simulink model "BiT_Template"  (R2025a)
settings: Solver=FixedStepDiscrete  StartTime=0.0  StopTime=Inf  FixedStep=0.005  RelTol=1e-3
StopFcn:
  | user_confirmed = true;
  | disp('Gestoppt?!')
  | 
  | % stop(t);
  | % delete(t);
  | 
  | %% Switch to Config Mode
  | %Tc3_AI.sysManager.ActivateConfiguration();
  | %
  | % Tc3_AI.SwitchToConfig('local')
  | %
  | % %save Solution
  | % Tc3_AI.SaveSolution();
  | %
  | % %% Close Aktive VS Instance
  | % Tc3_AI.closeVsInstance();
libraries: slpidlib x1
settings Model: SimulationMode=external  Creator=clemensm  LastModifiedBy=Lenard
settings OptimizationCC: LocalBlockOutputs=off
settings RTWCC: SystemTargetFile=TwinCatGrt.tlc  GenCodeOnly=on  GenerateMakefile=off  TemplateMakefile=tcgrt_msbuild.tmf  TargetLang=C++  Description=TwinCAT GRT Target
settings STFCustomTargetCC: SystemTargetFile=TwinCatGrt.tlc  TargetLangStandard=C++11 (ISO)  MultiwordLength=2048.0  DynamicStringBufferSize=256.0  ConcurrentExecutionCompliant=on  CombineOutputUpdateFcns=on  CodeInterfacePackaging=Reusable function  CPPClassGenCompliant=on  GRTInterface=off  GenerateAllocFcn=on  TcCom_DWorkReadOnly=on  TcProject_InstallPlcLibrary=off  TcProject_CLanguageStandard=Default  TcProject_PlcVarPrefixes=PVOID=p | BOOL=b | BOOL32=b | DATE=d | TIME_OF_DATE=td | TIME=t | LTIME=t | GUID=n  TcProject_PreferIntOverLong=off  TcPlcFb_OemLicenses=$<Project:OemLicenses>  TcCom_OutputCreateSymbols=on  TcCom_AccessLockState=Auto  TcProject_PublishTcUMx86=off  TcProject_PublishTcRTx64=on  TcPlcFb_ExtModeRtAllowExecutionCommands=off  TcCom_TcComWrapperFbProperties=off  TcProject_PublishTcOSARMv7M=off  TcCom_GroupIcon=$<TE140x:Icon>  TcCom_ModuleIcon=$<TE140x:Icon>  TcCom_ExecutionInfoParam=on  TcCom_CallerVerification=Default  TcProject_PublishTcRTx86=on  TcProject_CreateScopedEnums=Auto  TcCom_ExtModeRtWaitForStart=off  TcProject_TmxInstall=on  TcProject_Description=TwinCAT executable file, generated by TwinCAT $<ModuleGenerator:ProductId>  TcCom_ParametersReadOnly=off  TcCom_GroupDisplayName=$<GroupName>  TcProject_MaxVisibleArrayElements=200U  TcProject_ClassFactoryName=$<Project:Name>  TcCom_TcComWrapperFb=off  TcCom_UpdateExceptionHandling=CallerExceptions  TcProject_UseStaticStlString=off  TcCom_BlockIoReadOnly=on  TcCom_Legacy_ModuleBuildInfoParam=on  TcProject_UseCodeInfoExporter=on  TcProject_ProjectDir=C:\TwinCAT\3.1\CustomConfig\Modules\Ctrl_only  TcCom_ExtModeRtAllowForParameterChange=on  TcProject_GenerateStructDutsWithDefaultValues=Auto  TcProject_PublishTcOSx64=off  TcCom_OnlineChangeRestoreDataAreas=off  TcCom_BlockDiagramVariableAccess=AssignToParent  TcProject_LibraryCategories=$<VendorName>  TcProject_DeployRestart=off  TcProject_PublishTcOSARMv8A=off  TcProject_PublishPlatformtoolset=Auto  TcProject_UseIntrinsics=on  TcCom_ExecutionSequence=UpdateBeforeOutputMapping  TcCom_TcComWrapperFbPropertyMonitoring=NoMonitoring  TcProject_SignWithTwinCatCertificate=inherit default  TcProject_LowestCompatibleTcBuild=$<TwinCAT:Version:BUILD>  TcCom_StrictAccessLock=on  TcCom_ContStateDataAccess=Internal DataArea  TcCom_ExecutionInfoOutput=off  TcCom_OemLicenses=$<Project:OemLicenses>  TcCom_Generate=on  TcProject_ForceRebuildForPublish=off  TcProject_CppLanguageStandard=Default  TcProject_EnableNewPlatforms=off  TcCom_BlockDiagramDebugInfoExport=on  TcCom_StepSizeAdaptation=RequireMatchingTaskCycleTime  TcCom_InitExceptionHandling=CallerExceptions  TcProject_BuildWithWdk=inherit default  TcProject_VendorIcon=$<TE140x:Icon>  TcCom_InputReadOnly=off  TcCom_BlockIoDataAccess=Internal DataArea  TcProject_StaticStlStringCapacity=Auto  TcProject_ProductName=$<ModuleGenerator:ProductId> $<ModuleGenerator:Version:MAJOR.MINOR>  TcCom_DataStoreDataAccess=None  TcCom_InputInitValues=off  TcProject_IncrementVersion=Revision  TcProject_GenerateVsSolution=No  TcProject_Publish=on  TcProject_DataExchangeModulesVersion=$<ModuleGenerator:DataExchange:Version>  TcProject_BuildSystem=Auto  TcProject_Versioning=Versioned  TcCom_ExtendSignalResolution=on  TcCom_ResolveMaskedSubsystems=on  TcProject_SignTwinCatCertName=MCI_2024_OEM.tccert  TcProject_PublishParallel=on  TcPlcFb_Generate=off  TcCom_BlockIoCreateSymbols=on  TcCom_DWorkDataAccess=Internal DataArea  TcProject_VersionSrc=$<LatestTMFile>  TcProject_Verbosity=Normal  TcPlcFb_MonitorExecutionTime=off  TcPlcFb_UpdateExceptionHandling=CallerExceptions  TcProject_CoderCppNamespace=coder  TcCom_DWorkCreateSymbols=on  TcPlcFb_ExtModeRtWaitForStart=off  TcCom_AllowDataAreaForSharedData=off  TcCom_ParametersDataAccess=Internal DataArea  TcProject_UseTmxExtension=Auto  TcProject_DrvFileVersion=$<VersionFromFile>  TcCom_GlobalParamDefaultSharing=Define  TcCom_ParametersInitValues=on  TcCom_OutputReadOnly=on  TcProject_GeneratePlcLibrary=off  TcCom_ContStateCreateSymbols=on  TcCom_MonitorExecutionTime=off  TcProject_PublishTcUMx64=off  TcProject_PreferToolArchitectureX64=on  TcCom_GroupName=TE140x|Simulink Modules  TcCom_BlockDiagramExport=on  TcCom_ExecuteModelCode=on  TcProject_CreateUniqueEnumItemNames=off  TcProject_PublishConfiguration=Release  TcCom_ExtModeRtAllowExecutionCommands=on  TcProject_PublishTcOSARMv7A=off  TcProject_UseDescriptorCodeType=on  TcCom_ContStateReadOnly=on  TcCom_ParametersCreateSymbols=on  TcPlcFb_InitExceptionHandling=CallerExceptions  TcCom_ModuleCaller=CyclicTask  TcCom_OnlineChange=off  TcCom_InputDataAccess=Input Destination DataArea  TcCom_InputCreateSymbols=on  TcProject_DrvProductVersion=$<DrvFileVersion>  TcPlcFb_ExtModeRtAllowForParameterChange=off  TcCom_VariableSymbolMapping=Identical  TcCom_DataStoreReadOnly=off  TcCom_OriginalIoBlockNames=off  TcProject_UseCodeDescriptor=on  TcProject_VendorName=TE140x Module Vendor  TcProject_Copyright=Copyright $<VendorName> $<LocalDateTime:%Y>  TcProject_Generate=on  TcCom_DataStoreCreateSymbols=on  TcCom_OutputDataAccess=Output Source DataArea  TcProject_LibCatPath=$<Project:Dir>\$<Project:Name>.libcat.xml  TcProject_UseNativeBlockDiagramExport=off  TcProject_UseDataExchangeModules=off
settings GRTTargetCC: ExtMode=on  ExtModeMexFile=TcExtModeClient  MultiInstanceErrorCode=None  TargetLangStandard=C++11 (ISO)  ParMdlRefBuildCompliant=off  CompOptLevelCompliant=off  MatFileLogging=off  CodeInterfacePackaging=Reusable function  GenerateAllocFcn=on  UseToolchainInfoCompliant=off

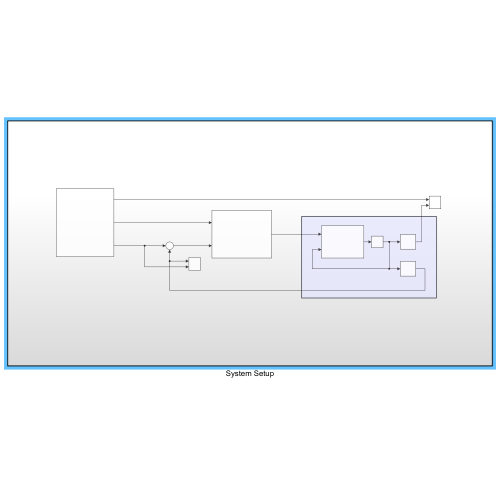
[thumbnail: Simulink's stored preview of the top-level diagram]
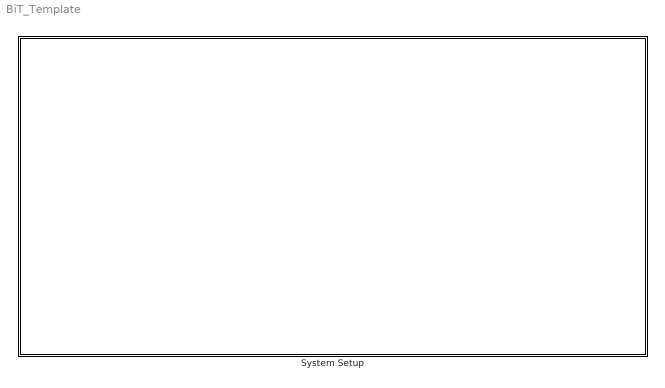
== system BiT_Template ==
  System Setup : Subsystem

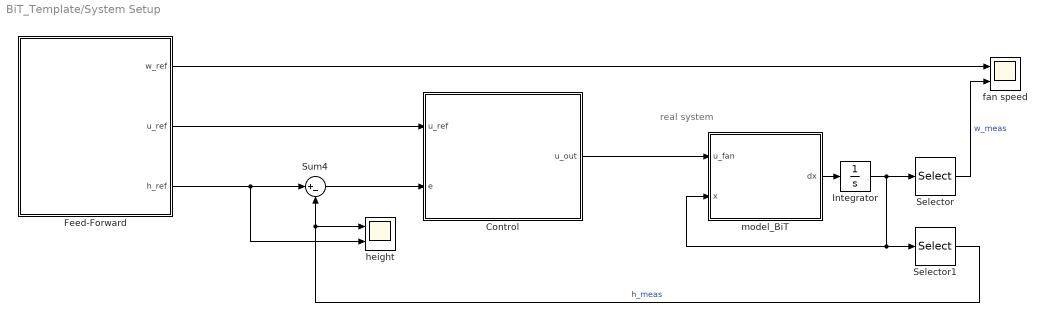
== system BiT_Template/System Setup ==
  note: real system
  Control : Subsystem
  Feed-Forward : Subsystem
  Integrator : Integrator
  Selector : Selector  InputPortWidth=3  IndexOptions=Index vector (dialog)  Indices=3  OutputSizes=1
  Selector1 : Selector  InputPortWidth=3  IndexOptions=Index vector (dialog)  Indices=1  OutputSizes=1
  Sum4 : Sum  Inputs=|+-
  fan speed : Scope  NumInputPorts=2
      settings: TimeSpan=60  ActiveDisplayYMinimum=4277  ActiveDisplayYMaximum=4777
  height : Scope  NumInputPorts=2
      settings: TimeSpan=60  ActiveDisplayYMinimum=0.11937  ActiveDisplayYMaximum=0.40562  DataLoggingVariableName=ScopeData2
  model_BiT : MATLAB Function  TreatAsAtomicUnit=on
  wires:
  Selector1/1 -> height/1, Sum4/2  "h_meas"
  Selector/1 -> fan speed/2  "w_meas"
  model_BiT/1(dx) -> Integrator/1
  Integrator/1 -> Selector/1, Selector1/1, model_BiT/2(x)
  Feed-Forward/3(h_ref) -> height/2, Sum4/1
  Feed-Forward/1(w_ref) -> fan speed/1
  Feed-Forward/2(u_ref) -> Control/1(u_ref)
  Sum4/1 -> Control/2(e)
  Control/1(u_out) -> model_BiT/1(u_fan)

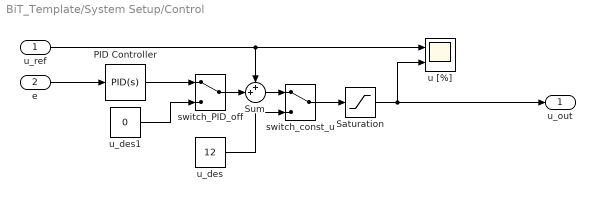
== system BiT_Template/System Setup/Control ==
  u_ref : Inport
  e : Inport  Port=2
  PID Controller : slpidlib/PID Controller  Controller=PID  Form=Parallel  TimeDomain=Continuous-time  UseExternalTs=off  SampleTime=-1  IntegratorMethod=Forward Euler  FilterMethod=Forward Euler  ControllerParametersSource=internal  P=1  I=1  UseKiTs=off  D=0  UseExternalDerivativeSource=off  N=100  UseFilter=on  TunerSelectOption=Transfer Function Based (PID Tuner App)  InitialConditionSource=internal  InitialConditionForIntegrator=0  InitialConditionForFilter=0  DifferentiatorICPrevScaledInput=0  ExternalReset=none  TrackingMode=off  Kt=1  LimitOutput=off  SatLimitsSource=internal  UpperSaturationLimit=inf  LowerSaturationLimit=-inf  LinearizeAsGain=on  AntiWindupMode=none  Kb=1  LimitIntegrator=off  UpperIntegratorSaturationLimit=inf  LowerIntegratorSaturationLimit=-inf  POutMin=[]  POutMax=[]  IOutMin=[]  IOutMax=[]  DOutMin=[]  DOutMax=[]  NOutMin=[]  NOutMax=[]  SumOutMin=[]  SumOutMax=[]  SaturationOutMin=[]  SaturationOutMax=[]  PParamMin=[]  PParamMax=[]  IParamMin=[]  IParamMax=[]  DParamMin=[]  DParamMax=[]  NParamMin=[]  NParamMax=[]  KbParamMin=[]  KbParamMax=[]  KtParamMin=[]  KtParamMax=[]  KbOutMin=[]  KbOutMax=[]  KtOutMin=[]  KtOutMax=[]  IntegratorOutMin=[]  IntegratorOutMax=[]  FilterOutMin=[]  FilterOutMax=[]  SumI1OutMin=[]  SumI1OutMax=[]  SumI2OutMin=[]  SumI2OutMax=[]  SumI3OutMin=[]  SumI3OutMax=[]  SumI4OutMin=[]  SumI4OutMax=[]  SumDOutMin=[]  SumDOutMax=[]  DifferentiatorOutMin=[]  DifferentiatorOutMax=[]  FilterDiffOutCoefMin=[]  FilterDiffOutCoefMax=[]  ReciprocalOutMin=[]  ReciprocalOutMax=[]  SumDenOutMin=[]  SumDenOutMax=[]  SumNumOutMin=[]  SumNumOutMax=[]  DivideOutMin=[]  DivideOutMax=[]  UdiffTsProdOutMin=[]  UdiffTsProdOutMax=[]  NTsProdOutMin=[]  NTsProdOutMax=[]  UintegralTsProdOutMin=[]  UintegralTsProdOutMax=[]  UngainTsProdOutMin=[]  UngainTsProdOutMax=[]  ClampingZeroOutDataTypeStr=Inherit: Inherit via back propagation  ClampingZeroOutMin=[]  ClampingZeroOutMax=[]  FilterDenConstantOutDataTypeStr=Inherit: Inherit via back propagation  FilterDenConstantOutMin=[]  FilterDenConstantOutMax=[]  PCopyOutDataTypeStr=Inherit: Inherit via back propagation  PCopyOutMin=[]  PCopyOutMax=[]  NCopyOutDataTypeStr=Inherit: Inherit via back propagation  NCopyOutMin=[]  NCopyOutMax=[]  IntegratorContinuousStateAttributes=''  IntegratorStateMustResolveToSignalObject=off  IntegratorRTWStateStorageClass=Auto  FilterContinuousStateAttributes=''  FilterStateMustResolveToSignalObject=off  FilterRTWStateStorageClass=Auto  ParallelPVariant=InternalParameters  IdealPVariant=Disabled  IVariant=InternalParameters  DVariant=InternalParameters  IntegratorVariant=Continuous  SatVariant=Disabled  AWVariant=Passthrough  PCopyVariant=Disabled  TRVariant=Disabled  FdbkBlocksVariant=Forward  IdealPFdbkVariant=Disabled  SatFdbkVariant=Disabled  DerivativeFilterVariant=ContFilter  NVariant=InternalParameters  NCopyVariant=Disabled  FilterICVariant=InternalICsFilter  IntegratorICVariant=InternalICs  ExternalResetVariant=Disabled  TRSumVariant=Passthrough  SumFdbkVariant=Disabled  SumVariant=Sum_PID  TsampFilterVariant=InternalTs  TsampNgainVariant=Passthrough  TsampIntegralVariant=Disabled_SignalSpec  ExternalSaturationOutDataTypeStr=Inherit: Same as second input  DerivativeSourceVariant=ErrorSignal  PreIntVariant=InternalPreInt
  Saturation : Saturate  UpperLimit=100  LowerLimit=0
  Sum : Sum  Inputs=++|
  switch_PID_off : ManualSwitch
  switch_const_u : ManualSwitch
  u [%] : Scope  NumInputPorts=2
      settings: TimeSpan=60  ActiveDisplayYMinimum=-141.60185  ActiveDisplayYMaximum=179.99898
  u_des : Constant  Value=12
  u_des1 : Constant  Value=0
  u_out : Outport
  wires:
  u_des/1 -> switch_const_u/2
  Saturation/1 -> u_out/1, u [%]/2
  e/1 -> PID Controller/1
  switch_const_u/1 -> Saturation/1
  u_ref/1 -> u [%]/1, Sum/1
  Sum/1 -> switch_const_u/1
  PID Controller/1 -> switch_PID_off/1
  switch_PID_off/1 -> Sum/2
  u_des1/1 -> switch_PID_off/2

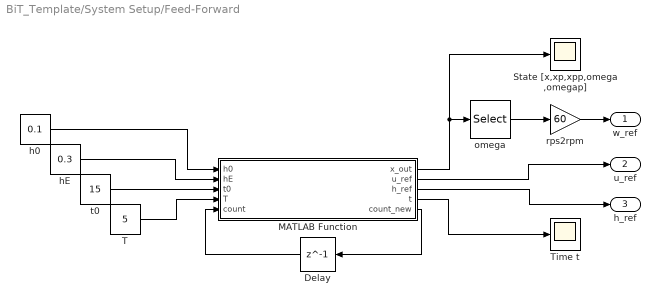
== system BiT_Template/System Setup/Feed-Forward ==
  Delay : Delay  DelayLength=1
  MATLAB Function : MATLAB Function  TreatAsAtomicUnit=on
  State [x,xp,xpp,omega,omegap] : Scope
      settings: TimeSpan=60  ActiveDisplayYMinimum=-34.55818  ActiveDisplayYMaximum=92.49741
  T : Constant  Value=5
  Time t : Scope
      settings: ActiveDisplayYMinimum=-17.36  ActiveDisplayYMaximum=-4.86
  h0 : Constant  Value=0.1
  hE : Constant  Value=0.3
  omega : Selector  InputPortWidth=5  IndexOptions=Index vector (dialog)  Indices=4  OutputSizes=1
  rps2rpm : Gain  Gain=60
  t0 : Constant  Value=15
  w_ref : Outport
  u_ref : Outport  Port=2
  h_ref : Outport  Port=3
  wires:
  h0/1 -> MATLAB Function/1(h0)
  omega/1 -> rps2rpm/1
  MATLAB Function/4(t) -> Time t/1
  T/1 -> MATLAB Function/4(T)
  t0/1 -> MATLAB Function/3(t0)
  Delay/1 -> MATLAB Function/5(count)
  MATLAB Function/5(count_new) -> Delay/1
  hE/1 -> MATLAB Function/2(hE)
  MATLAB Function/1(x_out) -> State [x,xp,xpp,omega,omegap]/1, omega/1
  MATLAB Function/2(u_ref) -> u_ref/1
  MATLAB Function/3(h_ref) -> h_ref/1
  rps2rpm/1 -> w_ref/1

== matlab function BiT_Template/System Setup/model_BiT ==
  data: u_fan input; dx output; x input
function dx = model_BiT(u_fan, x)
%#codegen
% Plant "Ball in Tube" mit realer Lüfterkennlinie:
%   u_fan  : Duty in %
%   x      : [z; zdot; w]  (w in rpm)
%   dx     : [zdot; zddot; wdot]

% --- Parameter 
% Lüfter-Dynamik
tau_omega = 1.4;                 % [s] Zeitkonstante PT1
%k_omega = 39.125;

% Statische Kennlinie (Messpunkte)  u[%] -> w[rpm]
% -> 0% = 4000 rpm (Leerlauf), 10% = 4570 rpm, 90% = 7700 rpm
u_bp  = [0    10    90    100];  % [%]
w_tab = [4000 4570  7700  7700]; % [rpm]


% Ball-/Rohr-Parameter
a1 = 7.08e-4;
a2 = 1.11;
a3 = 9.81;

% Zustände 
z    = x(1);     % [m]
zdot = x(2);     % [m/s]
w    = x(3);     % [rpm]

% Balldynamik
zddot = (a1*w - a2*zdot)^2 - a3;

% --- Lüfter: statische Kennlinie + PT1-Dynamik 
% Eingangsgrenzen (SIM: 0..100 %; für reale HW ggf. 10..90 %)
u = max(0, min(100, u_fan));                     % clamp 0..100 %

% Statischer Sollwert der Drehzahl aus LUT
% (linear; bei Bedarf 'pchip' für glattere Kurve)
w_ss = interp1(u_bp, w_tab, u, 'linear', 'extrap');

% PT1 auf den statischen Sollwert
wdot = (w_ss - w) / tau_omega;                   % [rpm/s]
%wdot = (k_omega*(u_fan) - w)/tau_omega;

% --- Ausgabe 
dx = [zdot; zddot; wdot];
end

== matlab function BiT_Template/System Setup/Feed-Forward/MATLAB Function ==
  data: x_out output; u_ref output; h0 input; hE input; t0 input; T input; h_ref output; t output; count input; count_new output
function [x_out,u_ref,h_ref,t,count_new] = feed_forward(h0,hE,t0,T,count)

count_new = count+1;
dT = 0.005;
t = count_new*dT-t0;

% Parameter



% Calculate Trajectory

xp_ref = 0;
xpp_ref = 0;
xppp_ref = 0;

if t<0
    x_ref = h0;
elseif t>T
    x_ref = hE;
else
    x_ref = h0; % Trajectory has to be implemented!
end

% Equations:
omega = 0; % equation for omega
omega_p = 0; % equation for omega
u = 0; % equation for omega

h_ref = x_ref;
u_ref = u; 
x_out = [x_ref,xp_ref,xpp_ref,omega,omega_p]';
end
